simulink model "dspqdemo"  (Simulink 5.0)
settings: Solver=FixedStepDiscrete  StartTime=0.0  StopTime=inf  RelTol=1e-3
libraries: dspsrcs4 x3, simulink3 x2, dspbuff3 x1
settings Model: Creator=don  LastModifiedBy=mkhan  SaveTime=off  SaveOutput=off  LimitDataPoints=off  IntegerOverflowMsg=none  RTWOptions="-aEnforceIntegerDowncast=1 -aExtMode=0 -aFoldNonRolledExpr=1 -aForceParamTrailComments=0 -aGenRTModel=1 -aGenerateComments=1 -aGenerateReport=0 -aIgnoreCustomStorageClasses=1 -aIncHierarchyInIds=0 -aInlineInvariantSignals=0 -aLocalBlockOutputs=1 -aLogVarNameModifier=\"rt_\" -aRTWVerbose=1 -aRollThreshold=5 -aShowEliminatedStatements=1"  RTWRetainRTWFile=on  ExtModeTrigMode=oneshot  ExtModeArmWhenConnect=off  BlockReductionOpt=off  BooleanDataType=off

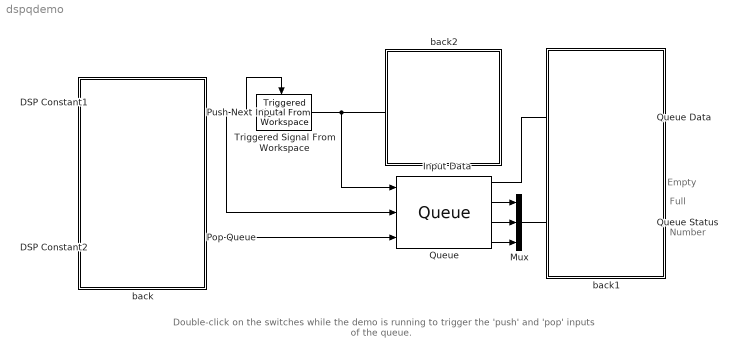
== system dspqdemo ==
  note: Number
  note: Full
  note: Empty
  note: Double-click on the switches while the demo is running
      | to trigger the 'push' and 'pop' inputs of the queue.
  DSP Constant1 : dspsrcs4/DSP Constant  Value=1  InterpretAs1D=on  SampleMode=Discrete  Ts=4  FramebasedOutput=off
  DSP Constant2 : dspsrcs4/DSP Constant  Value=0  InterpretAs1D=on  SampleMode=Discrete  Ts=4  FramebasedOutput=off
  Input Data : Display
      settings: Format=short
  Mux : Mux  Inputs=3
  Pop Queue : simulink3/Nonlinear/Manual Switch  sw=1  action=0
  Push Next Input : simulink3/Nonlinear/Manual Switch  sw=1  action=0
  Queue : dspbuff3/Queue  depth=3  trigger=Either edge  overflow=Warning  pes=Warning  eso=on  fso=on  nso=on  clr=off  clrOutport=on
  Queue Data : Display
      settings: Format=short
  Queue Status : Display
      settings: Format=short
  Triggered Signal From Workspace : dspsrcs4/Triggered Signal From Workspace  Signal=1:16  TriggerType=Either edge  ic=0  SamplesPerFrame=4  OutputAfterFinalValue=Setting To Zero
  back : Subsystem
      settings: RTWFcnNameOpts=Auto  RTWFileNameOpts=Auto
  back1 : Subsystem
      settings: RTWFcnNameOpts=Auto  RTWFileNameOpts=Auto
  back2 : Subsystem
      settings: RTWFcnNameOpts=Auto  RTWFileNameOpts=Auto
  wires:
  Pop Queue/1 -> Queue/3
  Queue/3 -> Mux/2
  Queue/2 -> Mux/1
  Queue/4 -> Mux/3
  Mux/1 -> Queue Status/1
  Push Next Input/1 -> Queue/2, Triggered Signal From Workspace/Trigger
  DSP Constant1/1 -> Pop Queue/1, Push Next Input/1
  DSP Constant2/1 -> Pop Queue/2, Push Next Input/2
  Queue/1 -> Queue Data/1
  Triggered Signal From Workspace/1 -> Input Data/1, Queue/1

== system dspqdemo/back ==

== system dspqdemo/back1 ==

== system dspqdemo/back2 ==
